simulink model "convert_SimBus"  (R2018b)
settings: configuration reference "Physics" (kept outside this file)
undefined symbols (not defined in the file or in its folder): TUMHealthStatus
settings Model: DataDictionary=convert_SimBus.sldd  PauseTimes=9.280  Creator=wischnewski  LastModifiedBy=ge34qer

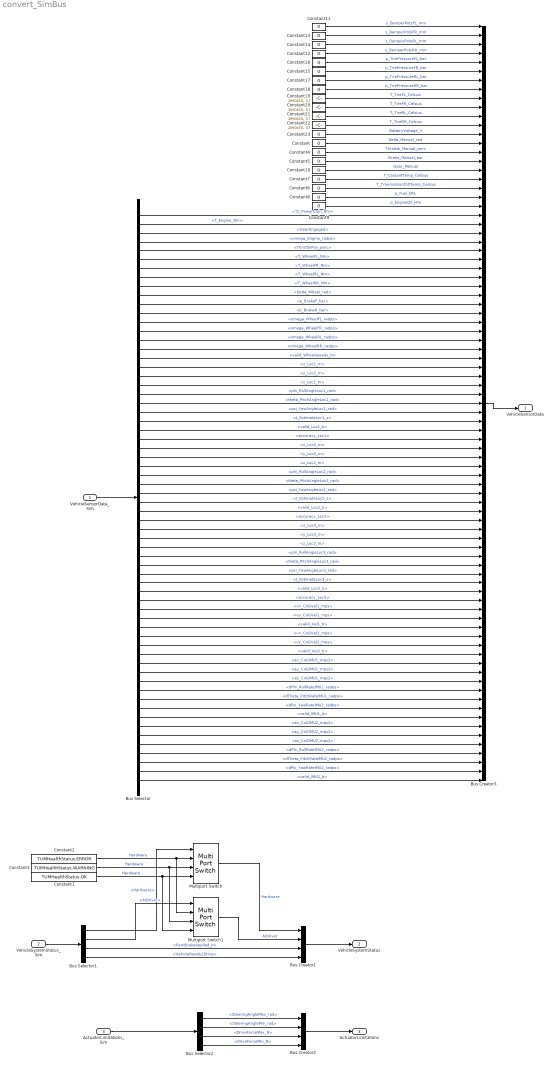
== system convert_SimBus ==
  VehicleSensorData_Sim : Inport  OutDataTypeStr=Bus: VehicleSensorData_Sim
  VehicleSystemStatus_Sim : Inport  Port=2  OutDataTypeStr=Bus: VehicleSystemStatus_Sim
  ActuatorLimitations_Sim : Inport  Port=3  OutDataTypeStr=Bus: ActuatorLimitations_Sim
  Bus Creator1 : BusCreator  Inputs=4  OutDataTypeStr=Bus: VehicleSystemStatus
  Bus Creator2 : BusCreator  Inputs=4  OutDataTypeStr=Bus: ActuatorLimitations
  Bus Creator3 : BusCreator  Inputs=85  OutDataTypeStr=Bus: VehicleSensorData
  Bus Selector : BusSelector  OutputSignals=Tz_Powertrain_Nm,T_Engine_Nm,GearEngaged,omega_Engine_radps,ThrottlePos_perc,T_WheelFL_Nm,T_WheelFR_Nm,T_WheelRL_Nm,T_WheelRR_Nm,Delta_Wheel_rad,p_BrakeF_bar,p_BrakeR_bar,omega_WheelFL_radps,omega_WheelFR_radps,omega_WheelRL_radps,omega_WheelRR_radps,valid_Wheelspeeds_b,x_Loc1_m,y_Loc1_m,z_Loc1_m,phi_RollAngleLoc1_rad,theta_PitchAngleLoc1_rad,psi_YawAngleLoc1_rad,t_EstimateLoc1_s,valid_Loc1_b,accuracy_Loc1,x_Loc2_m,y_Loc2_m,z_Loc2_m,phi_RollAngleLoc2_rad,theta_PitchAngleLoc2_rad,psi_YawAngleLoc2_rad,t_EstimateLoc2_s,valid_Loc2_b,accuracy_Loc2,x_Loc3_m,y_Loc3_m,z_Loc3_m,phi_RollAngleLoc3_rad,theta_PitchAngleLoc3_rad,psi_YawAngleLoc3_rad,t_EstimateLoc3_s,valid_Loc3_b,accuracy_Loc3,vx_CoGVel1_mps,vy_CoGVel1_mps,valid_Vel1_b,vx_CoGVel2_mps,vy_CoGVel2_mps,valid_Vel2_b,ax_CoGIMU1_mps2,ay_CoGIMU1_mps2,az_CoGIMU1_mps2,dPhi_RollRateIMU1_radps,dTheta_PitchRateIMU1_radps,dPsi_YawRateIMU1_radps,valid_IMU1_b,ax_CoGIMU2_mps2,ay_CoGIMU2_mps2,az_CoGIMU2_mps2,dPhi_RollRateIMU2_radps,dTheta_PitchRateIMU2_radps,dPsi_YawRateIMU2_radps,valid_IMU2_b
  Bus Selector1 : BusSelector  OutputSignals=Hardware,AIDriver,ParkBrakeApplied_b,VehicleReady2Drive
  Bus Selector2 : BusSelector  OutputSignals=SteeringAngleMax_rad,SteeringAngleMin_rad,DriveForceMax_N,DriveForceMin_N
  Constant{,4..18,23} (17 alike) : Constant  Value=0
  Constant1 : Constant  Value=TUMHealthStatus.OK
  Constant{19..22} (4 alike) : Constant  Value=zeros(4, 1)
  Constant2 : Constant  Value=TUMHealthStatus.ERROR
  Constant3 : Constant  Value=TUMHealthStatus.WARNING
  Multiport Switch : MultiPortSwitch  DataPortOrder=Zero-based contiguous  zeroidx=on
  Multiport Switch1 : MultiPortSwitch  DataPortOrder=Zero-based contiguous  zeroidx=on
  VehicleSensorData : Outport  OutDataTypeStr=Bus: VehicleSensorData
  VehicleSystemStatus : Outport  Port=2  OutDataTypeStr=Bus: VehicleSystemStatus
  ActuatorLimitations : Outport  Port=3  OutDataTypeStr=Bus: ActuatorLimitations
  wires:
  VehicleSystemStatus_Sim/1 -> Bus Selector1/1
  Bus Selector1/2 -> Multiport Switch1/1  "<AIDriver>"
  Bus Creator2/1 -> ActuatorLimitations/1
  Multiport Switch/1 -> Bus Creator1/1  "Hardware"
  Constant3/1 -> Multiport Switch1/3, Multiport Switch/3  "Hardware"
  Constant2/1 -> Multiport Switch1/2, Multiport Switch/2  "Hardware"
  Constant1/1 -> Multiport Switch1/4, Multiport Switch/4  "Hardware"
  Bus Selector1/1 -> Multiport Switch/1  "<Hardware>"
  Bus Selector2/3 -> Bus Creator2/3  "<DriveForceMax_N>"
  Bus Creator1/1 -> VehicleSystemStatus/1
  Bus Selector1/4 -> Bus Creator1/4  "<VehicleReady2Drive>"
  ActuatorLimitations_Sim/1 -> Bus Selector2/1
  Bus Creator3/1 -> VehicleSensorData/1
  Bus Selector1/3 -> Bus Creator1/3  "<ParkBrakeApplied_b>"
  Bus Selector2/4 -> Bus Creator2/4  "<DriveForceMin_N>"
  Multiport Switch1/1 -> Bus Creator1/2  "AIDriver"
  Bus Selector2/1 -> Bus Creator2/1  "<SteeringAngleMax_rad>"
  Bus Selector2/2 -> Bus Creator2/2  "<SteeringAngleMin_rad>"
  VehicleSensorData_Sim/1 -> Bus Selector/1
  Bus Selector/4 -> Bus Creator3/25  "<omega_Engine_radps>"
  Bus Selector/3 -> Bus Creator3/24  "<GearEngaged>"
  Bus Selector/1 -> Bus Creator3/22  "<Tz_Powertrain_Nm>"
  Bus Selector/6 -> Bus Creator3/27  "<T_WheelFL_Nm>"
  Bus Selector/7 -> Bus Creator3/28  "<T_WheelFR_Nm>"
  Bus Selector/8 -> Bus Creator3/29  "<T_WheelRL_Nm>"
  Bus Selector/9 -> Bus Creator3/30  "<T_WheelRR_Nm>"
  Bus Selector/10 -> Bus Creator3/31  "<Delta_Wheel_rad>"
  Bus Selector/11 -> Bus Creator3/32  "<p_BrakeF_bar>"
  Bus Selector/12 -> Bus Creator3/33  "<p_BrakeR_bar>"
  Bus Selector/13 -> Bus Creator3/34  "<omega_WheelFL_radps>"
  Bus Selector/14 -> Bus Creator3/35  "<omega_WheelFR_radps>"
  Bus Selector/15 -> Bus Creator3/36  "<omega_WheelRL_radps>"
  Bus Selector/16 -> Bus Creator3/37  "<omega_WheelRR_radps>"
  Bus Selector/17 -> Bus Creator3/38  "<valid_Wheelspeeds_b>"
  Bus Selector/18 -> Bus Creator3/39  "<x_Loc1_m>"
  Bus Selector/19 -> Bus Creator3/40  "<y_Loc1_m>"
  Bus Selector/20 -> Bus Creator3/41  "<z_Loc1_m>"
  Bus Selector/21 -> Bus Creator3/42  "<phi_RollAngleLoc1_rad>"
  Bus Selector/22 -> Bus Creator3/43  "<theta_PitchAngleLoc1_rad>"
  Bus Selector/23 -> Bus Creator3/44  "<psi_YawAngleLoc1_rad>"
  Bus Selector/24 -> Bus Creator3/45  "<t_EstimateLoc1_s>"
  Bus Selector/25 -> Bus Creator3/46  "<valid_Loc1_b>"
  Bus Selector/26 -> Bus Creator3/47  "<accuracy_Loc1>"
  Bus Selector/27 -> Bus Creator3/48  "<x_Loc2_m>"
  Bus Selector/28 -> Bus Creator3/49  "<y_Loc2_m>"
  Bus Selector/29 -> Bus Creator3/50  "<z_Loc2_m>"
  Bus Selector/30 -> Bus Creator3/51  "<phi_RollAngleLoc2_rad>"
  Bus Selector/31 -> Bus Creator3/52  "<theta_PitchAngleLoc2_rad>"
  Bus Selector/32 -> Bus Creator3/53  "<psi_YawAngleLoc2_rad>"
  Bus Selector/33 -> Bus Creator3/54  "<t_EstimateLoc2_s>"
  Bus Selector/34 -> Bus Creator3/55  "<valid_Loc2_b>"
  Bus Selector/35 -> Bus Creator3/56  "<accuracy_Loc2>"
  Bus Selector/45 -> Bus Creator3/66  "<vx_CoGVel1_mps>"
  Bus Selector/46 -> Bus Creator3/67  "<vy_CoGVel1_mps>"
  Bus Selector/47 -> Bus Creator3/68  "<valid_Vel1_b>"
  Bus Selector/48 -> Bus Creator3/69  "<vx_CoGVel2_mps>"
  Bus Selector/49 -> Bus Creator3/70  "<vy_CoGVel2_mps>"
  Bus Selector/50 -> Bus Creator3/71  "<valid_Vel2_b>"
  Bus Selector/51 -> Bus Creator3/72  "<ax_CoGIMU1_mps2>"
  Bus Selector/52 -> Bus Creator3/73  "<ay_CoGIMU1_mps2>"
  Bus Selector/53 -> Bus Creator3/74  "<az_CoGIMU1_mps2>"
  Bus Selector/54 -> Bus Creator3/75  "<dPhi_RollRateIMU1_radps>"
  Bus Selector/55 -> Bus Creator3/76  "<dTheta_PitchRateIMU1_radps>"
  Bus Selector/56 -> Bus Creator3/77  "<dPsi_YawRateIMU1_radps>"
  Bus Selector/57 -> Bus Creator3/78  "<valid_IMU1_b>"
  Bus Selector/58 -> Bus Creator3/79  "<ax_CoGIMU2_mps2>"
  Bus Selector/59 -> Bus Creator3/80  "<ay_CoGIMU2_mps2>"
  Bus Selector/60 -> Bus Creator3/81  "<az_CoGIMU2_mps2>"
  Bus Selector/61 -> Bus Creator3/82  "<dPhi_RollRateIMU2_radps>"
  Bus Selector/62 -> Bus Creator3/83  "<dTheta_PitchRateIMU2_radps>"
  Bus Selector/63 -> Bus Creator3/84  "<dPsi_YawRateIMU2_radps>"
  Bus Selector/64 -> Bus Creator3/85  "<valid_IMU2_b>"
  Bus Selector/2 -> Bus Creator3/23  "<T_Engine_Nm>"
  Bus Selector/5 -> Bus Creator3/26  "<ThrottlePos_perc>"
  Bus Selector/36 -> Bus Creator3/57  "<x_Loc3_m>"
  Bus Selector/37 -> Bus Creator3/58  "<y_Loc3_m>"
  Bus Selector/38 -> Bus Creator3/59  "<z_Loc3_m>"
  Bus Selector/39 -> Bus Creator3/60  "<phi_RollAngleLoc3_rad>"
  Bus Selector/40 -> Bus Creator3/61  "<theta_PitchAngleLoc3_rad>"
  Bus Selector/41 -> Bus Creator3/62  "<psi_YawAngleLoc3_rad>"
  Bus Selector/42 -> Bus Creator3/63  "<t_EstimateLoc3_s>"
  Bus Selector/43 -> Bus Creator3/64  "<valid_Loc3_b>"
  Bus Selector/44 -> Bus Creator3/65  "<accuracy_Loc3>"
  Constant/1 -> Bus Creator3/14  "Delta_Manual_rad"
  Constant9/1 -> Bus Creator3/21  "p_EngineOil_kPa"
  Constant8/1 -> Bus Creator3/20  "p_Fuel_kPa"
  Constant7/1 -> Bus Creator3/18  "T_CoolantTemp_Celsius"
  Constant6/1 -> Bus Creator3/19  "T_TranmissionOilTtemp_Celsius"
  Constant10/1 -> Bus Creator3/17  "Gear_Manual"
  Constant5/1 -> Bus Creator3/16  "Brake_Manual_bar"
  Constant4/1 -> Bus Creator3/15  "Throttle_Manual_perc"
  Constant11/1 -> Bus Creator3/1  "s_DamperPotsFL_mm"
  Constant13/1 -> Bus Creator3/2  "s_DamperPotsFR_mm"
  Constant14/1 -> Bus Creator3/3  "s_DamperPotsRL_mm"
  Constant12/1 -> Bus Creator3/4  "s_DamperPotsRR_mm"
  Constant16/1 -> Bus Creator3/5  "p_TirePressureFL_bar"
  Constant15/1 -> Bus Creator3/6  "p_TirePressureFR_bar"
  Constant17/1 -> Bus Creator3/7  "p_TirePressureRL_bar"
  Constant18/1 -> Bus Creator3/8  "p_TirePressureRR_bar"
  Constant19/1 -> Bus Creator3/9  "T_TireFL_Celsius"
  Constant20/1 -> Bus Creator3/10  "T_TireFR_Celsius"
  Constant21/1 -> Bus Creator3/11  "T_TireRL_Celsius"
  Constant22/1 -> Bus Creator3/12  "T_TireRR_Celsius"
  Constant23/1 -> Bus Creator3/13  "BatteryVoltage_V"
